simulink model "LPN_CVS_LVAD"  (R2014b)
settings: Solver=ode23s  StartTime=0.0  StopTime=15  FixedStep=0.01  RelTol=1e-2
values from neighbouring files (symbols this model uses):
  Cao = 0.08    [LPN_CVS_LVAD_Parameters.mat]
  Ccorat = 0.004    [LPN_CVS_LVAD_Parameters.mat]
  Ccorvn = 0.093    [LPN_CVS_LVAD_Parameters.mat]
  Cpa = 0.18    [LPN_CVS_LVAD_Parameters.mat]
  Cpart = 3.8    [LPN_CVS_LVAD_Parameters.mat]
  Cpvn = 20.5    [LPN_CVS_LVAD_Parameters.mat]
  CQao = 300    [LPN_CVS_LVAD_Parameters.mat]
  CQmi = 400    [LPN_CVS_LVAD_Parameters.mat]
  CQpa = 350    [LPN_CVS_LVAD_Parameters.mat]
  CQtri = 400    [LPN_CVS_LVAD_Parameters.mat]
  CsartLB = 1.9    [LPN_CVS_LVAD_Parameters.mat]
  CsartUB = 0.5    [LPN_CVS_LVAD_Parameters.mat]
  CsvnLB = 15    [LPN_CVS_LVAD_Parameters.mat]
  CsvnUB = 4    [LPN_CVS_LVAD_Parameters.mat]
  EedLA = 0.2125    [LPN_CVS_LVAD_Parameters.mat]
  EedRA = 0.1575    [LPN_CVS_LVAD_Parameters.mat]
  EmaxLA = 0.45    [LPN_CVS_LVAD_Parameters.mat]
  EmaxLV = 2.8    [LPN_CVS_LVAD_Parameters.mat]
  EmaxRA = 0.225    [LPN_CVS_LVAD_Parameters.mat]
  EmaxRV = 0.727    [LPN_CVS_LVAD_Parameters.mat]
  LV_Pd_alpha = 0.064    [LPN_CVS_LVAD_Parameters.mat]
  LV_Pd_beta = 2.5    [LPN_CVS_LVAD_Parameters.mat]
  LV_Pd_kappa = 0.033    [LPN_CVS_LVAD_Parameters.mat]
  Rao = 0.003    [LPN_CVS_LVAD_Parameters.mat]
  Rcorat = 26.25    [LPN_CVS_LVAD_Parameters.mat]
  Rcorvn = 8.75    [LPN_CVS_LVAD_Parameters.mat]
  Rpa = 0.002    [LPN_CVS_LVAD_Parameters.mat]
  Rpart = 0.31    [LPN_CVS_LVAD_Parameters.mat]
  Rpvn = 0.075    [LPN_CVS_LVAD_Parameters.mat]
  RsartLB = 2.3    [LPN_CVS_LVAD_Parameters.mat]
  RsartUB = 3.57    [LPN_CVS_LVAD_Parameters.mat]
  RsvnLB = 0.05    [LPN_CVS_LVAD_Parameters.mat]
  RsvnUB = 0.33    [LPN_CVS_LVAD_Parameters.mat]
  RV_Pd_alpha = 0.047    [LPN_CVS_LVAD_Parameters.mat]
  RV_Pd_beta = 2.5    [LPN_CVS_LVAD_Parameters.mat]
  RV_Pd_kappa = 0.028    [LPN_CVS_LVAD_Parameters.mat]
  V0ao = 112    [LPN_CVS_LVAD_Parameters.mat]
  V0ao_us = 101    [LPN_CVS_LVAD_Parameters.mat]
  V0corat = 6    [LPN_CVS_LVAD_Parameters.mat]
  V0corat_us = 5    [LPN_CVS_LVAD_Parameters.mat]
  V0corvn = 10    [LPN_CVS_LVAD_Parameters.mat]
  V0corvn_us = 9    [LPN_CVS_LVAD_Parameters.mat]
  V0LA = 22    [LPN_CVS_LVAD_Parameters.mat]
  V0LA_us = 5    [LPN_CVS_LVAD_Parameters.mat]
  V0LV = 95    [LPN_CVS_LVAD_Parameters.mat]
  V0LV_us = 5    [LPN_CVS_LVAD_Parameters.mat]
  V0pa = 78    [LPN_CVS_LVAD_Parameters.mat]
  V0pa_us = 77    [LPN_CVS_LVAD_Parameters.mat]
  V0part = 211    [LPN_CVS_LVAD_Parameters.mat]
  V0part_us = 91    [LPN_CVS_LVAD_Parameters.mat]
  V0pvn = 388    [LPN_CVS_LVAD_Parameters.mat]
  V0pvn_us = 168    [LPN_CVS_LVAD_Parameters.mat]
  V0RA = 20    [LPN_CVS_LVAD_Parameters.mat]
  V0RA_us = 5    [LPN_CVS_LVAD_Parameters.mat]
  V0RV = 125    [LPN_CVS_LVAD_Parameters.mat]
  V0RV_us = 10    [LPN_CVS_LVAD_Parameters.mat]
  V0sart_usLB = 91    [LPN_CVS_LVAD_Parameters.mat]
  V0sart_usUB = 39    [LPN_CVS_LVAD_Parameters.mat]
  V0sartLB = 301    [LPN_CVS_LVAD_Parameters.mat]
  V0sartUB = 87    [LPN_CVS_LVAD_Parameters.mat]
  V0svn_usLB = 385    [LPN_CVS_LVAD_Parameters.mat]
  V0svn_usUB = 165    [LPN_CVS_LVAD_Parameters.mat]
  V0svnLB = 477    [LPN_CVS_LVAD_Parameters.mat]
  V0svnUB = 220    [LPN_CVS_LVAD_Parameters.mat]
libraries: simulink x6
settings Model: Creator=Michael  LastModifiedBy=Michael
settings SolverCC: ZeroCrossAlgorithm=Adaptive
settings DataIOCC: MaxDataPoints=100

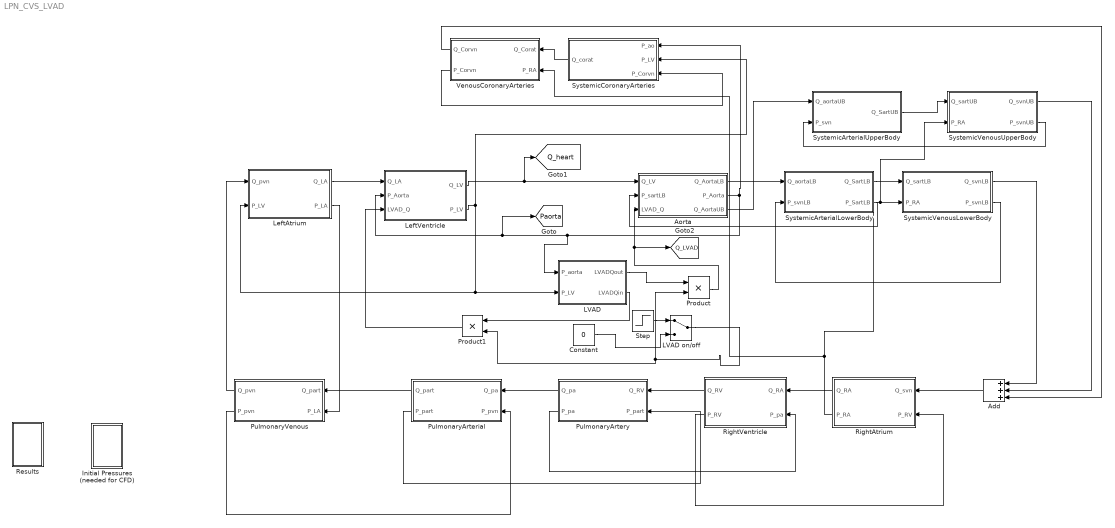
== system LPN_CVS_LVAD ==
  Add : Sum  Inputs=+++
  Aorta : Subsystem
  Constant : Constant  Value=0
  Initial Pressures (needed for CFD) : Subsystem
  LVAD : Subsystem
  LVAD on/off : ManualSwitch
  LeftAtrium : Subsystem
  LeftVentricle : Subsystem
  Product : Product
  Product1 : Product
  PulmonaryArterial : Subsystem
  PulmonaryArtery : Subsystem
  PulmonaryVenous : Subsystem
  Results : Subsystem
  RightAtrium : Subsystem
  RightVentricle : Subsystem
  Step : Step  Time=8  SampleTime=0
  SystemicArterialLowerBody : Subsystem
  SystemicArterialUpperBody : Subsystem
  SystemicCoronaryArteries : Subsystem
  SystemicVenousLowerBody : Subsystem
  SystemicVenousUpperBody : Subsystem
  VenousCoronaryArteries : Subsystem
  tag scope: Paorta=global, Q_LVAD=global, Q_heart=global
  wires:
  LeftVentricle/1(Q_LV) -> [Q_heart], Aorta/1(Q_LV)
  Aorta/1(Q_AortaLB) -> SystemicArterialLowerBody/1(Q_aortaLB)
  Aorta/2(P_Aorta) -> SystemicCoronaryArteries/1(P_ao), LVAD/1(P_aorta), [Paorta], LeftVentricle/2(P_Aorta)
  SystemicVenousLowerBody/2(P_svnLB) -> SystemicArterialLowerBody/2(P_svnLB)
  SystemicArterialLowerBody/1(Q_SartLB) -> SystemicVenousLowerBody/1(Q_sartLB)
  LeftAtrium/1(Q_LA) -> LeftVentricle/1(Q_LA)
  RightAtrium/1(Q_RA) -> RightVentricle/1(Q_RA)
  RightVentricle/1(Q_RV) -> PulmonaryArtery/1(Q_RV)
  PulmonaryArtery/2(P_pa) -> RightVentricle/2(P_pa)
  PulmonaryArterial/2(P_part) -> PulmonaryArtery/2(P_part)
  RightAtrium/2(P_RA) -> VenousCoronaryArteries/2(P_RA), SystemicVenousUpperBody/2(P_RA), SystemicVenousLowerBody/2(P_RA)
  PulmonaryArtery/1(Q_pa) -> PulmonaryArterial/1(Q_pa)
  PulmonaryArterial/1(Q_part) -> PulmonaryVenous/1(Q_part)
  PulmonaryVenous/2(P_pvn) -> PulmonaryArterial/2(P_pvn)
  LeftAtrium/2(P_LA) -> PulmonaryVenous/2(P_LA)
  PulmonaryVenous/1(Q_pvn) -> LeftAtrium/1(Q_pvn)
  SystemicArterialUpperBody/1(Q_SartUB) -> SystemicVenousUpperBody/1(Q_sartUB)
  SystemicVenousUpperBody/2(P_svnUB) -> SystemicArterialUpperBody/2(P_svn)
  Add/1 -> RightAtrium/1(Q_svn)
  SystemicVenousLowerBody/1(Q_svnLB) -> Add/1
  SystemicVenousUpperBody/1(Q_svnUB) -> Add/2
  SystemicArterialLowerBody/2(P_SartLB) -> Aorta/2(P_sartLB)
  Aorta/3(Q_AortaUB) -> SystemicArterialUpperBody/1(Q_aortaUB)
  RightVentricle/2(P_RV) -> RightAtrium/2(P_RV)
  LeftVentricle/2(P_LV) -> LVAD/2(P_LV), LeftAtrium/2(P_LV), SystemicCoronaryArteries/2(P_LV)
  SystemicCoronaryArteries/1(Q_corat) -> VenousCoronaryArteries/1(Q_Corat)
  VenousCoronaryArteries/2(P_Corvn) -> SystemicCoronaryArteries/3(P_Corvn)
  VenousCoronaryArteries/1(Q_Corvn) -> Add/3
  Constant/1 -> LVAD on/off/2
  Step/1 -> LVAD on/off/1
  LVAD/1(LVADQout) -> Product/1
  LVAD on/off/1 -> Product/2, Product1/2
  Product/1 -> [Q_LVAD], Aorta/3(LVAD_Q)
  Product1/1 -> LeftVentricle/3(LVAD_Q)
  LVAD/2("LVADQin ") -> Product1/1

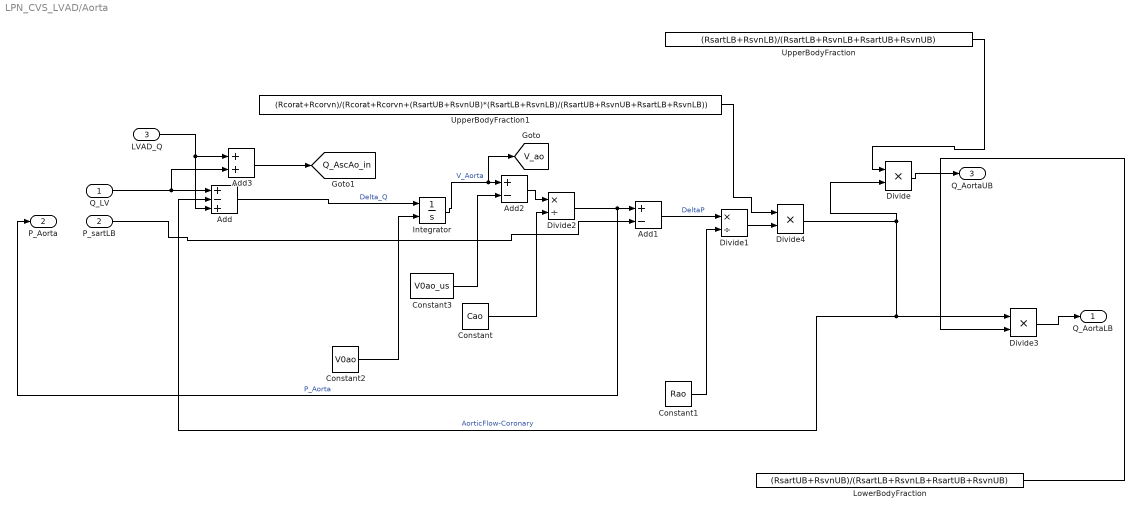
== system LPN_CVS_LVAD/Aorta ==
  Q_LV : Inport
  P_sartLB : Inport  Port=2
  LVAD_Q : Inport  Port=3
  Add : Sum  Inputs=+-+
  Add1 : Sum  Inputs=+-
  Add2 : Sum  Inputs=+-
  Add3 : Sum
  Constant : Constant  Value=Cao
  Constant1 : Constant  Value=Rao
  Constant2 : Constant  Value=V0ao
  Constant3 : Constant  Value=V0ao_us
  Divide : Product  Inputs=**
  Divide1 : Product  Inputs=*/
  Divide2 : Product  Inputs=*/
  Divide3 : Product  Inputs=**
  Divide4 : Product  Inputs=**
  Integrator : Integrator  InitialConditionSource=external
  LowerBodyFraction : Constant  Value=(RsartUB+RsvnUB)/(RsartLB+RsvnLB+RsartUB+RsvnUB)
  UpperBodyFraction : Constant  Value=(RsartLB+RsvnLB)/(RsartLB+RsvnLB+RsartUB+RsvnUB)
  UpperBodyFraction1 : Constant  Value=(Rcorat+Rcorvn)/(Rcorat+Rcorvn+(RsartUB+RsvnUB)*(RsartLB+RsvnLB)/(RsartUB+RsvnUB+RsartLB+RsvnLB))
  Q_AortaLB : Outport
  P_Aorta : Outport  Port=2
  Q_AortaUB : Outport  Port=3
  tag scope: Q_AscAo_in=global, V_ao=global
  wires:
  Add/1 -> Integrator/1  "Delta_Q"
  Constant1/1 -> Divide1/2
  Add1/1 -> Divide1/1  "DeltaP"
  Constant/1 -> Divide2/2
  P_sartLB/1 -> Add1/2
  Q_LV/1 -> Add3/2, Add/1
  Integrator/1 -> [V_ao], Add2/1  "V_Aorta"
  Constant2/1 -> Integrator/2
  Add2/1 -> Divide2/1
  Divide2/1 -> P_Aorta/1, Add1/1  "P_Aorta"
  Constant3/1 -> Add2/2
  Divide/1 -> Q_AortaUB/1
  Divide3/1 -> Q_AortaLB/1
  LowerBodyFraction/1 -> Divide3/2
  UpperBodyFraction/1 -> Divide/1
  UpperBodyFraction1/1 -> Divide4/1
  Divide1/1 -> Divide4/2
  Divide4/1 -> Add/2, Divide3/1, Divide/2  "AorticFlow-Coronary"
  LVAD_Q/1 -> Add3/1, Add/3
  Add3/1 -> [Q_AscAo_in]

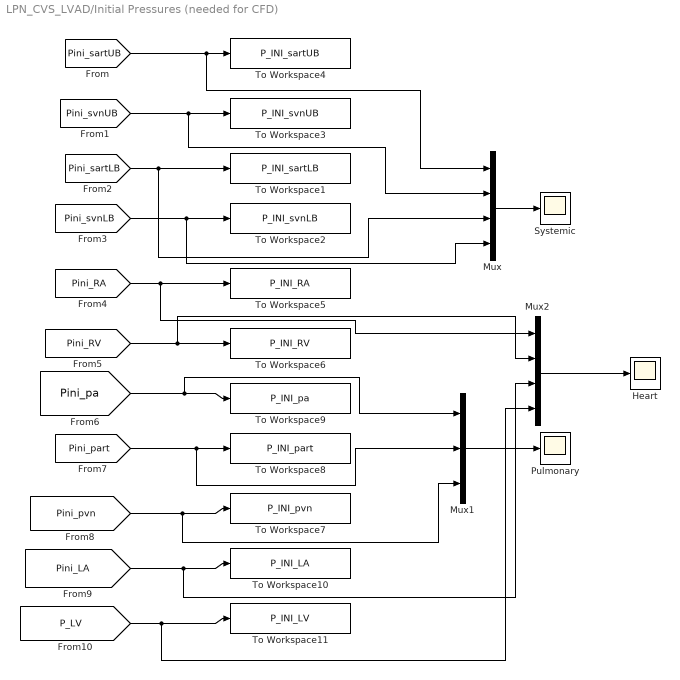
== system LPN_CVS_LVAD/Initial Pressures (needed for CFD) ==
  Heart : Scope
      settings: SaveName=ScopeData18
  Mux : Mux
  Mux1 : Mux  Inputs=3
  Mux2 : Mux
  Pulmonary : Scope
      settings: SaveName=ScopeData17
  Systemic : Scope
      settings: SaveName=ScopeData16
  To Workspace1 : ToWorkspace  VariableName=P_INI_sartLB  SampleTime=-1
  To Workspace10 : ToWorkspace  VariableName=P_INI_LA  SampleTime=-1
  To Workspace11 : ToWorkspace  VariableName=P_INI_LV  SampleTime=-1
  To Workspace2 : ToWorkspace  VariableName=P_INI_svnLB  SampleTime=-1
  To Workspace3 : ToWorkspace  VariableName=P_INI_svnUB  SampleTime=-1
  To Workspace4 : ToWorkspace  VariableName=P_INI_sartUB  SampleTime=-1
  To Workspace5 : ToWorkspace  VariableName=P_INI_RA  SampleTime=-1
  To Workspace6 : ToWorkspace  VariableName=P_INI_RV  SampleTime=-1
  To Workspace7 : ToWorkspace  VariableName=P_INI_pvn  SampleTime=-1
  To Workspace8 : ToWorkspace  VariableName=P_INI_part  SampleTime=-1
  To Workspace9 : ToWorkspace  VariableName=P_INI_pa  SampleTime=-1
  wires:
  [Pini_sartUB] -> Mux/1, To Workspace4/1
  [Pini_svnUB] -> Mux/2, To Workspace3/1
  [Pini_sartLB] -> Mux/3, To Workspace1/1
  [Pini_svnLB] -> Mux/4, To Workspace2/1
  [Pini_RA] -> Mux2/1, To Workspace5/1
  [Pini_RV] -> Mux2/2, To Workspace6/1
  [Pini_pa] -> Mux1/1, To Workspace9/1
  [Pini_part] -> Mux1/2, To Workspace8/1
  [Pini_pvn] -> Mux1/3, To Workspace7/1
  [Pini_LA] -> Mux2/3, To Workspace10/1
  [P_LV] -> Mux2/4, To Workspace11/1
  Mux1/1 -> Pulmonary/1
  Mux/1 -> Systemic/1
  Mux2/1 -> Heart/1

== system LPN_CVS_LVAD/LVAD ==
  P_aorta : Inport
  P_LV : Inport  Port=2
  Add2 : Sum  Inputs=+-
  Outlet Cannula : Subsystem
  PumpPerformance : Subsystem
  R_can_in : Gain  Gain=0.05
  Scope : Scope
      settings: SaveName=ScopeData24
  Scope1 : Scope
      settings: SaveName=ScopeData32
  LVADQout : Outport
  "LVADQin " : Outport  Port=2
  wires:
  P_aorta/1 -> Outlet Cannula/2(P_aorta)
  Outlet Cannula/2(LVADQout) -> LVADQout/1
  P_LV/1 -> Add2/1
  R_can_in/1 -> Add2/2
  PumpPerformance/1(LVADQin) -> Scope1/1, "LVADQin "/1, R_can_in/1, Outlet Cannula/1(LVADQin)
  Add2/1 -> PumpPerformance/1(P_can_in), Scope/1
  Outlet Cannula/1(P_can_out) -> PumpPerformance/2(P_can_out)

== system LPN_CVS_LVAD/LeftAtrium ==
  Q_pvn : Inport
  P_LV : Inport  Port=2
  Add : Sum  Inputs=+-
  Add2 : Sum  Inputs=+-
  AtrialElastance : Subsystem
  Constant2 : Constant  Value=V0LA
  Integrator : Integrator  InitialConditionSource=external
  Mitral Valve : Subsystem
  Product : Product
  Repeating Sequence : simulink/Sources/Repeating Sequence  rep_seq_t=time  rep_seq_y=e_a
  V0LA_US : Constant  Value=V0LA_us
  Q_LA : Outport
  P_LA : Outport  Port=2
  tag scope: Pini_LA=global, V_la=global
  wires:
  Q_pvn/1 -> Add2/1
  Add/1 -> Product/1
  V0LA_US/1 -> Add/2  "V0"
  Add2/1 -> Integrator/1  "Q_compliance"
  Integrator/1 -> [V_la], Add/1  "V_LV"
  Product/1 -> Mitral Valve/1(P_LA), [Pini_LA], P_LA/1  "P_LV(t)"
  Repeating Sequence/1 -> AtrialElastance/1(e_a)  "e_a"
  AtrialElastance/1(E(t)) -> Product/2
  Constant2/1 -> Integrator/2
  Mitral Valve/1(Q_LA) -> Q_LA/1, Add2/2
  P_LV/1 -> Mitral Valve/2(P_LV)

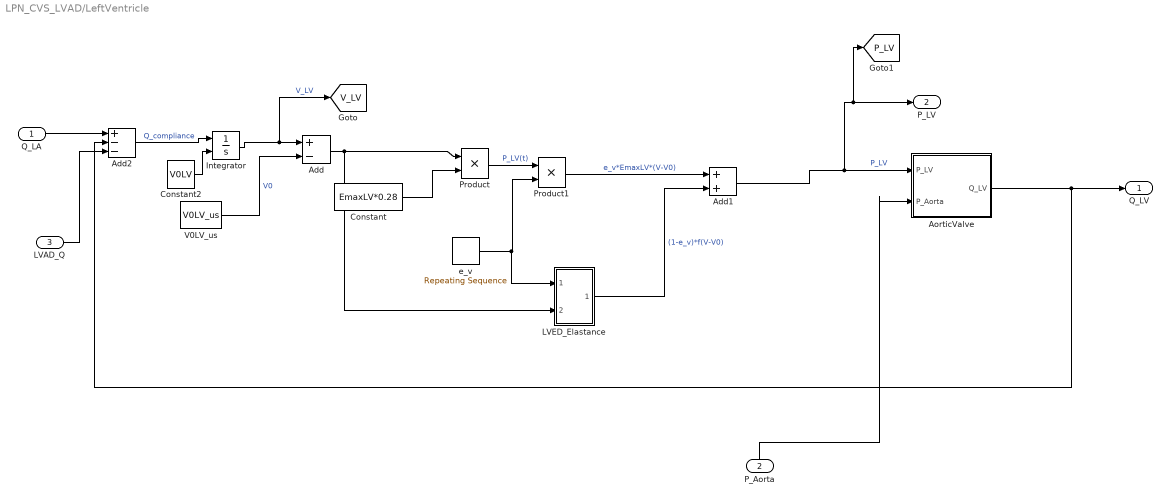
== system LPN_CVS_LVAD/LeftVentricle ==
  Q_LA : Inport
  P_Aorta : Inport  Port=2
  LVAD_Q : Inport  Port=3
  Add : Sum  Inputs=+-
  Add1 : Sum
  Add2 : Sum  Inputs=+--
  AorticValve : Subsystem
  Constant : Constant  Value=EmaxLV*0.28
  Constant2 : Constant  Value=V0LV
  Integrator : Integrator  InitialConditionSource=external
  LVED_Elastance : Subsystem
  Product : Product
  Product1 : Product
  V0LV_us : Constant  Value=V0LV_us
  e_v : simulink/Sources/Repeating Sequence  rep_seq_t=time  rep_seq_y=e_v
  Q_LV : Outport
  P_LV : Outport  Port=2
  tag scope: P_LV=global, V_LV=global
  wires:
  Q_LA/1 -> Add2/1
  Add/1 -> LVED_Elastance/2(V-V0), Product/1
  V0LV_us/1 -> Add/2  "V0"
  Add2/1 -> Integrator/1  "Q_compliance"
  Integrator/1 -> [V_LV], Add/1  "V_LV"
  Constant2/1 -> Integrator/2
  AorticValve/1(Q_LV) -> Add2/2, Q_LV/1
  P_Aorta/1 -> AorticValve/2(P_Aorta)
  Constant/1 -> Product/2
  Product/1 -> Product1/1  "P_LV(t)"
  e_v/1 -> LVED_Elastance/1(e_v), Product1/2
  Product1/1 -> Add1/1  "e_v*EmaxLV*(V-V0)"
  Add1/1 -> [P_LV], P_LV/1, AorticValve/1(P_LV)  "P_LV"
  LVED_Elastance/1(Eed) -> Add1/2  "(1-e_v)*f(V-V0)"
  LVAD_Q/1 -> Add2/3

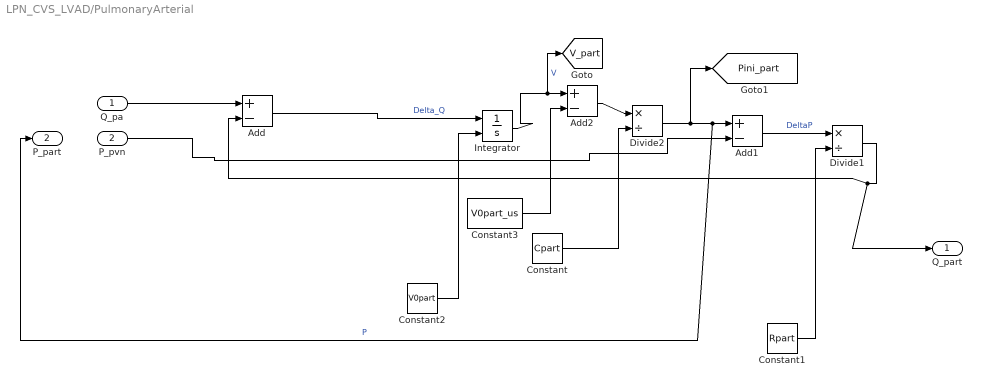
== system LPN_CVS_LVAD/PulmonaryArterial ==
  Q_pa : Inport
  P_pvn : Inport  Port=2
  Add : Sum  Inputs=+-
  Add1 : Sum  Inputs=+-
  Add2 : Sum  Inputs=+-
  Constant : Constant  Value=Cpart
  Constant1 : Constant  Value=Rpart
  Constant2 : Constant  Value=V0part
  Constant3 : Constant  Value=V0part_us
  Divide1 : Product  Inputs=*/
  Divide2 : Product  Inputs=*/
  Integrator : Integrator  InitialConditionSource=external
  Q_part : Outport
  P_part : Outport  Port=2
  tag scope: Pini_part=global, V_part=global
  wires:
  Divide1/1 -> Add/2, Q_part/1
  Add/1 -> Integrator/1  "Delta_Q"
  Constant1/1 -> Divide1/2
  Add1/1 -> Divide1/1  "DeltaP"
  Constant/1 -> Divide2/2
  P_pvn/1 -> Add1/2
  Q_pa/1 -> Add/1
  Integrator/1 -> [V_part], Add2/1  "V"
  Constant2/1 -> Integrator/2
  Add2/1 -> Divide2/1
  Divide2/1 -> [Pini_part], P_part/1, Add1/1  "P"
  Constant3/1 -> Add2/2

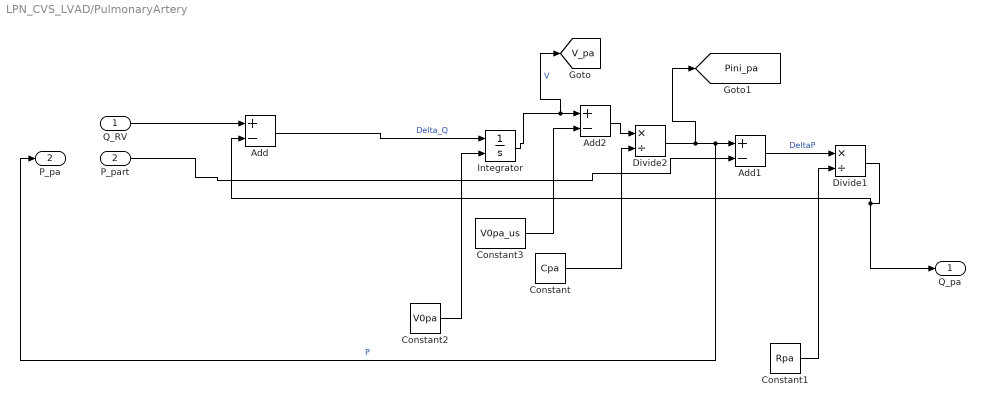
== system LPN_CVS_LVAD/PulmonaryArtery ==
  Q_RV : Inport
  P_part : Inport  Port=2
  Add : Sum  Inputs=+-
  Add1 : Sum  Inputs=+-
  Add2 : Sum  Inputs=+-
  Constant : Constant  Value=Cpa
  Constant1 : Constant  Value=Rpa
  Constant2 : Constant  Value=V0pa
  Constant3 : Constant  Value=V0pa_us
  Divide1 : Product  Inputs=*/
  Divide2 : Product  Inputs=*/
  Integrator : Integrator  InitialConditionSource=external
  Q_pa : Outport
  P_pa : Outport  Port=2
  tag scope: Pini_pa=global, V_pa=global
  wires:
  Divide1/1 -> Add/2, Q_pa/1
  Add/1 -> Integrator/1  "Delta_Q"
  Constant1/1 -> Divide1/2
  Add1/1 -> Divide1/1  "DeltaP"
  Constant/1 -> Divide2/2
  P_part/1 -> Add1/2
  Q_RV/1 -> Add/1
  Integrator/1 -> [V_pa], Add2/1  "V"
  Constant2/1 -> Integrator/2
  Add2/1 -> Divide2/1
  Divide2/1 -> [Pini_pa], P_pa/1, Add1/1  "P"
  Constant3/1 -> Add2/2

== system LPN_CVS_LVAD/PulmonaryVenous ==
  Q_part : Inport
  P_LA : Inport  Port=2
  Add : Sum  Inputs=+-
  Add1 : Sum  Inputs=+-
  Add2 : Sum  Inputs=+-
  Constant : Constant  Value=Cpvn
  Constant1 : Constant  Value=Rpvn
  Constant2 : Constant  Value=V0pvn
  Constant3 : Constant  Value=V0pvn_us  VectorParams1D=off
  Divide1 : Product  Inputs=*/
  Divide2 : Product  Inputs=*/
  Integrator : Integrator  InitialConditionSource=external
  Q_pvn : Outport
  P_pvn : Outport  Port=2
  tag scope: Pini_pvn=global, V_pvn=global
  wires:
  Divide1/1 -> Add/2, Q_pvn/1
  Add/1 -> Integrator/1  "Delta_Q"
  Constant1/1 -> Divide1/2
  Add1/1 -> Divide1/1  "DeltaP"
  Constant/1 -> Divide2/2
  P_LA/1 -> Add1/2
  Q_part/1 -> Add/1
  Integrator/1 -> [V_pvn], Add2/1  "V"
  Constant2/1 -> Integrator/2
  Add2/1 -> Divide2/1
  Divide2/1 -> [Pini_pvn], P_pvn/1, Add1/1  "P"
  Constant3/1 -> Add2/2

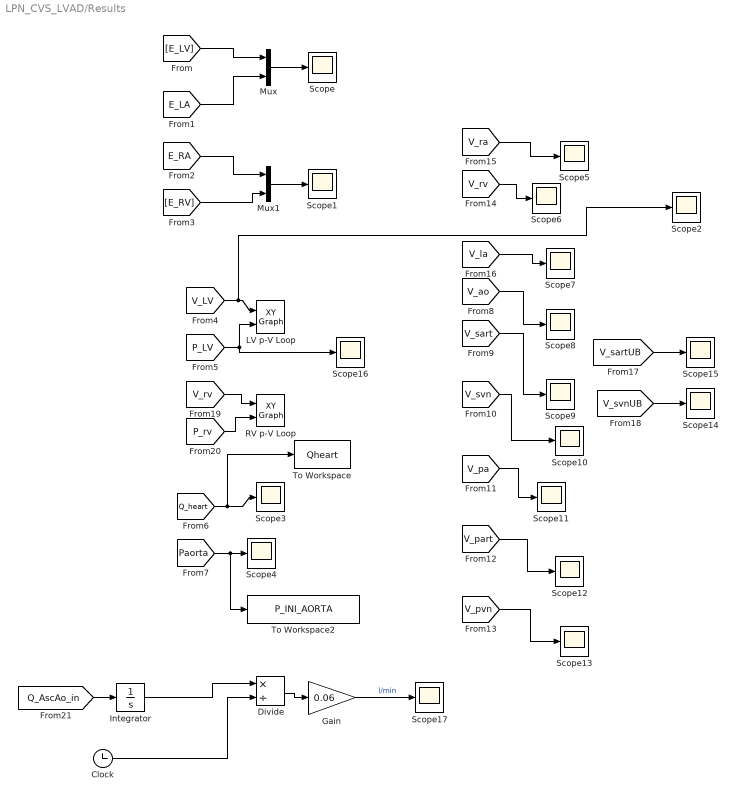
== system LPN_CVS_LVAD/Results ==
  Clock : Clock
  Divide : Product  Inputs=*/
  Gain : Gain  Gain=0.06
  Integrator : Integrator
  LV p-V Loop : simulink/Sinks/XY Graph  xmin=-1  xmax=200  ymin=-1  ymax=150  st=-1
  Mux : Mux  Inputs=2
  Mux1 : Mux  Inputs=2
  RV p-V Loop : simulink/Sinks/XY Graph  xmin=-1  xmax=150  ymin=-1  ymax=150  st=-1
  Scope{,1..17} (18 alike) : Scope
      Scope10 settings: SaveName=ScopeData12
      Scope11 settings: SaveName=ScopeData13
      Scope12 settings: YMin=240  YMax=330  SaveName=ScopeData14
      Scope13 settings: SaveName=ScopeData15
      Scope14 settings: SaveName=ScopeData21
      Scope15 settings: SaveName=ScopeData22
      Scope16 settings: SaveName=ScopeData20
      Scope17 settings: YMin=48  YMax=64  SaveName=ScopeData30
      Scope2 settings: SaveName=ScopeData4
      Scope3 settings: TimeRange=12.57889009793254  YMin=0  YMax=713.4020618556701  SaveName=ScopeData5
      Scope4 settings: SaveName=ScopeData6
      Scope5 settings: SaveName=ScopeData7
      Scope6 settings: SaveName=ScopeData8
      Scope7 settings: SaveName=ScopeData9
      Scope8 settings: SaveName=ScopeData10
      Scope9 settings: SaveName=ScopeData11
  To Workspace : ToWorkspace  VariableName=Qheart  SampleTime=-1
      settings: MaxDataPoints=100
  To Workspace2 : ToWorkspace  VariableName=P_INI_AORTA  SampleTime=-1
  wires:
  Mux1/1 -> Scope1/1
  Mux/1 -> Scope/1
  [E_LV] -> Mux/1
  [E_RA] -> Mux1/1
  [E_RV] -> Mux1/2
  [E_LA] -> Mux/2
  [V_LV] -> Scope2/1, LV p-V Loop/1
  [P_LV] -> LV p-V Loop/2, Scope16/1
  [Q_heart] -> To Workspace/1, Scope3/1
  [V_ra] -> Scope5/1
  [V_rv] -> Scope6/1
  [V_la] -> Scope7/1
  [V_ao] -> Scope8/1
  [V_sart] -> Scope9/1
  [V_svn] -> Scope10/1
  [V_pa] -> Scope11/1
  [V_part] -> Scope12/1
  [V_pvn] -> Scope13/1
  [V_svnUB] -> Scope14/1
  [V_sartUB] -> Scope15/1
  [V_rv] -> RV p-V Loop/1
  [P_rv] -> RV p-V Loop/2
  [Paorta] -> To Workspace2/1, Scope4/1
  Integrator/1 -> Divide/1
  Clock/1 -> Divide/2
  Divide/1 -> Gain/1
  [Q_AscAo_in] -> Integrator/1
  Gain/1 -> Scope17/1  "l/min"

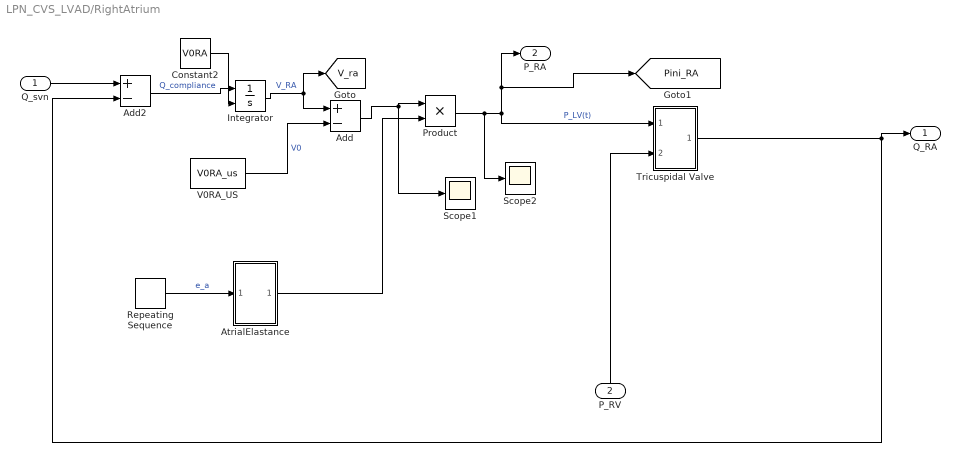
== system LPN_CVS_LVAD/RightAtrium ==
  Q_svn : Inport
  P_RV : Inport  Port=2
  Add : Sum  Inputs=+-
  Add2 : Sum  Inputs=+-
  AtrialElastance : Subsystem
  Constant2 : Constant  Value=V0RA
  Integrator : Integrator  InitialConditionSource=external
  Product : Product
  Repeating Sequence : simulink/Sources/Repeating Sequence  rep_seq_t=time  rep_seq_y=e_a
  Scope1 : Scope
      settings: SaveName=ScopeData2
  Scope2 : Scope
      settings: SaveName=ScopeData3
  Tricuspidal Valve : Subsystem
  V0RA_US : Constant  Value=V0RA_us
  Q_RA : Outport
  P_RA : Outport  Port=2
  tag scope: Pini_RA=global, V_ra=global
  wires:
  Q_svn/1 -> Add2/1
  Add/1 -> Product/1, Scope1/1
  V0RA_US/1 -> Add/2  "V0"
  Add2/1 -> Integrator/1  "Q_compliance"
  Integrator/1 -> [V_ra], Add/1  "V_RA"
  Product/1 -> Scope2/1, Tricuspidal Valve/1(P_RA), P_RA/1, [Pini_RA]  "P_LV(t)"
  Repeating Sequence/1 -> AtrialElastance/1(e_a)  "e_a"
  AtrialElastance/1(E(t)) -> Product/2
  Constant2/1 -> Integrator/2
  Tricuspidal Valve/1(Q_RV) -> Q_RA/1, Add2/2
  P_RV/1 -> Tricuspidal Valve/2(P_RV)

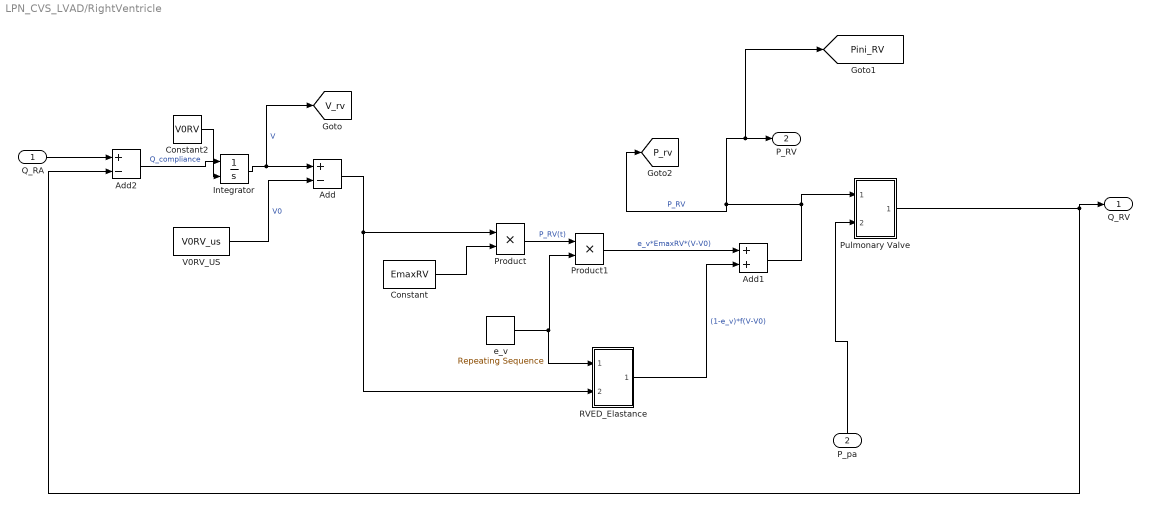
== system LPN_CVS_LVAD/RightVentricle ==
  Q_RA : Inport
  P_pa : Inport  Port=2
  Add : Sum  Inputs=+-
  Add1 : Sum
  Add2 : Sum  Inputs=+-
  Constant : Constant  Value=EmaxRV
  Constant2 : Constant  Value=V0RV
  Integrator : Integrator  InitialConditionSource=external
  Product : Product
  Product1 : Product
  Pulmonary Valve : Subsystem
  RVED_Elastance : Subsystem
  V0RV_US : Constant  Value=V0RV_us
  e_v : simulink/Sources/Repeating Sequence  rep_seq_t=time  rep_seq_y=e_v
  Q_RV : Outport
  P_RV : Outport  Port=2
  tag scope: P_rv=global, Pini_RV=global, V_rv=global
  wires:
  Q_RA/1 -> Add2/1
  V0RV_US/1 -> Add/2  "V0"
  Add2/1 -> Integrator/1  "Q_compliance"
  Integrator/1 -> [V_rv], Add/1  "V"
  Constant2/1 -> Integrator/2
  Pulmonary Valve/1(Q_RV) -> Q_RV/1, Add2/2
  P_pa/1 -> Pulmonary Valve/2(Ppa)
  Add/1 -> Product/1, RVED_Elastance/2(V-V0)
  Constant/1 -> Product/2
  Product/1 -> Product1/1  "P_RV(t)"
  e_v/1 -> RVED_Elastance/1(e_v), Product1/2
  Product1/1 -> Add1/1  "e_v*EmaxRV*(V-V0)"
  RVED_Elastance/1(Eed) -> Add1/2  "(1-e_v)*f(V-V0)"
  Add1/1 -> Pulmonary Valve/1(P_RV), [Pini_RV], P_RV/1, [P_rv]  "P_RV"

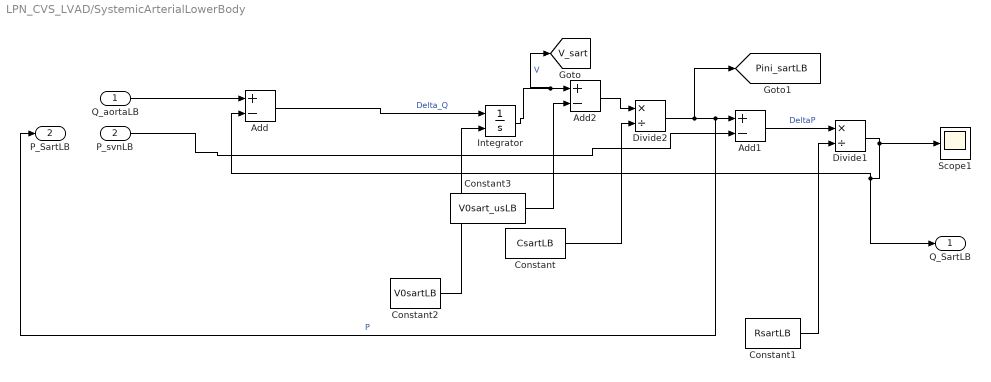
== system LPN_CVS_LVAD/SystemicArterialLowerBody ==
  Q_aortaLB : Inport
  P_svnLB : Inport  Port=2
  Add : Sum  Inputs=+-
  Add1 : Sum  Inputs=+-
  Add2 : Sum  Inputs=+-
  Constant : Constant  Value=CsartLB
  Constant1 : Constant  Value=RsartLB
  Constant2 : Constant  Value=V0sartLB
  Constant3 : Constant  Value=V0sart_usLB
  Divide1 : Product  Inputs=*/
  Divide2 : Product  Inputs=*/
  Integrator : Integrator  InitialConditionSource=external
  Scope1 : Scope
      settings: SaveName=ScopeData31
  Q_SartLB : Outport
  P_SartLB : Outport  Port=2
  tag scope: Pini_sartLB=global, V_sart=global
  wires:
  Divide1/1 -> Add/2, Q_SartLB/1, Scope1/1
  Add/1 -> Integrator/1  "Delta_Q"
  Constant1/1 -> Divide1/2
  Add1/1 -> Divide1/1  "DeltaP"
  Constant/1 -> Divide2/2
  P_svnLB/1 -> Add1/2
  Q_aortaLB/1 -> Add/1
  Integrator/1 -> [V_sart], Add2/1  "V"
  Constant2/1 -> Integrator/2
  Add2/1 -> Divide2/1
  Divide2/1 -> [Pini_sartLB], P_SartLB/1, Add1/1  "P"
  Constant3/1 -> Add2/2

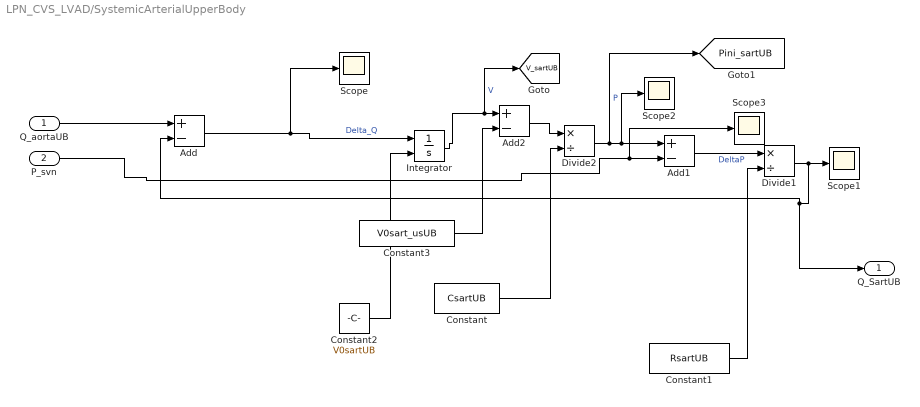
== system LPN_CVS_LVAD/SystemicArterialUpperBody ==
  Q_aortaUB : Inport
  P_svn : Inport  Port=2
  Add : Sum  Inputs=+-
  Add1 : Sum  Inputs=+-
  Add2 : Sum  Inputs=+-
  Constant : Constant  Value=CsartUB
  Constant1 : Constant  Value=RsartUB
  Constant2 : Constant  Value=V0sartUB
  Constant3 : Constant  Value=V0sart_usUB
  Divide1 : Product  Inputs=*/
  Divide2 : Product  Inputs=*/
  Integrator : Integrator  InitialConditionSource=external
  Scope{,1..3} (4 alike) : Scope
      Scope settings: SaveName=ScopeData26
      Scope1 settings: SaveName=ScopeData27
      Scope2 settings: SaveName=ScopeData28
      Scope3 settings: SaveName=ScopeData29
  Q_SartUB : Outport
  tag scope: Pini_sartUB=global, V_sartUB=global
  wires:
  Divide1/1 -> Add/2, Q_SartUB/1, Scope1/1
  Add/1 -> Scope/1, Integrator/1  "Delta_Q"
  Constant1/1 -> Divide1/2
  Add1/1 -> Divide1/1  "DeltaP"
  Constant/1 -> Divide2/2
  P_svn/1 -> Scope3/1, Add1/2
  Q_aortaUB/1 -> Add/1
  Integrator/1 -> [V_sartUB], Add2/1  "V"
  Constant2/1 -> Integrator/2
  Add2/1 -> Divide2/1
  Divide2/1 -> [Pini_sartUB], Scope2/1, Add1/1  "P"
  Constant3/1 -> Add2/2

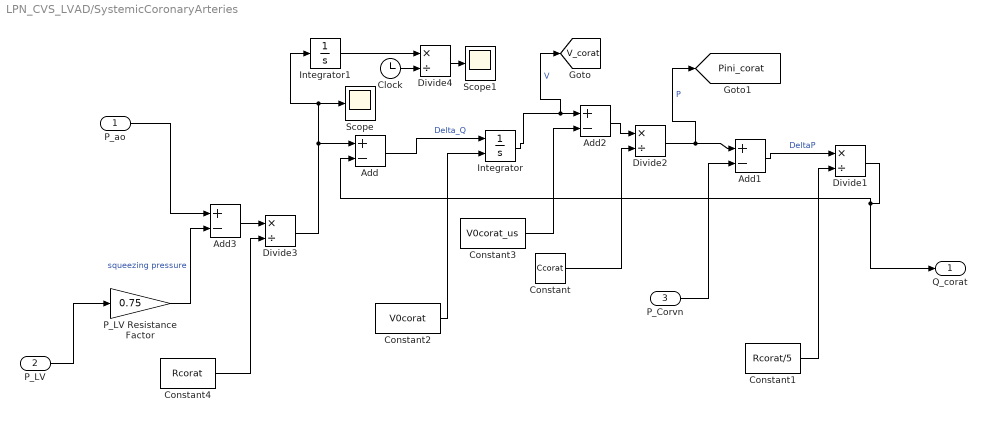
== system LPN_CVS_LVAD/SystemicCoronaryArteries ==
  P_ao : Inport
  P_LV : Inport  Port=2
  P_Corvn : Inport  Port=3
  Add{,1..3} (4 alike) : Sum  Inputs=+-
  Clock : Clock
  Constant : Constant  Value=Ccorat
  Constant1 : Constant  Value=Rcorat/5
  Constant2 : Constant  Value=V0corat
  Constant3 : Constant  Value=V0corat_us
  Constant4 : Constant  Value=Rcorat
  Divide{1..4} (4 alike) : Product  Inputs=*/
  Integrator : Integrator  InitialConditionSource=external
  Integrator1 : Integrator
  P_LV Resistance Factor : Gain  Gain=0.75
  Scope : Scope
      settings: YMin=-0.3  YMax=0  SaveName=ScopeData19
  Scope1 : Scope
      settings: YMin=-0.3  YMax=0  SaveName=ScopeData23
  Q_corat : Outport
  tag scope: Pini_corat=global, V_corat=global
  wires:
  Divide1/1 -> Add/2, Q_corat/1
  Add/1 -> Integrator/1  "Delta_Q"
  Constant1/1 -> Divide1/2
  Add1/1 -> Divide1/1  "DeltaP"
  Constant/1 -> Divide2/2
  P_LV/1 -> P_LV Resistance Factor/1
  Integrator/1 -> [V_corat], Add2/1  "V"
  Constant2/1 -> Integrator/2
  Add2/1 -> Divide2/1
  Divide2/1 -> [Pini_corat], Add1/1  "P"
  Constant3/1 -> Add2/2
  P_Corvn/1 -> Add1/2
  P_ao/1 -> Add3/1
  P_LV Resistance Factor/1 -> Add3/2  "squeezing pressure"
  Add3/1 -> Divide3/1
  Constant4/1 -> Divide3/2
  Divide3/1 -> Scope/1, Integrator1/1, Add/1
  Integrator1/1 -> Divide4/1
  Clock/1 -> Divide4/2
  Divide4/1 -> Scope1/1

== system LPN_CVS_LVAD/SystemicVenousLowerBody ==
  Q_sartLB : Inport
  P_RA : Inport  Port=2
  Add : Sum  Inputs=+-
  Add1 : Sum  Inputs=+-
  Add2 : Sum  Inputs=+-
  Constant : Constant  Value=CsvnLB
  Constant1 : Constant  Value=RsvnLB
  Constant2 : Constant  Value=V0svnLB
  Constant3 : Constant  Value=V0svn_usLB
  Divide1 : Product  Inputs=*/
  Divide2 : Product  Inputs=*/
  Integrator : Integrator  InitialConditionSource=external
  Q_svnLB : Outport
  P_svnLB : Outport  Port=2
  tag scope: Pini_svnLB=global, V_svn=global
  wires:
  Divide1/1 -> Add/2, Q_svnLB/1
  Add/1 -> Integrator/1  "Delta_Q"
  Constant1/1 -> Divide1/2
  Add1/1 -> Divide1/1  "DeltaP"
  Constant/1 -> Divide2/2
  P_RA/1 -> Add1/2
  Q_sartLB/1 -> Add/1
  Integrator/1 -> [V_svn], Add2/1  "V"
  Constant2/1 -> Integrator/2
  Add2/1 -> Divide2/1
  Divide2/1 -> [Pini_svnLB], P_svnLB/1, Add1/1  "P"
  Constant3/1 -> Add2/2

== system LPN_CVS_LVAD/SystemicVenousUpperBody ==
  Q_sartUB : Inport
  P_RA : Inport  Port=2
  Add : Sum  Inputs=+-
  Add1 : Sum  Inputs=+-
  Add2 : Sum  Inputs=+-
  Constant : Constant  Value=CsvnUB
  Constant1 : Constant  Value=RsvnUB
  Constant2 : Constant  Value=V0svnUB
  Constant3 : Constant  Value=V0svn_usUB
  Divide1 : Product  Inputs=*/
  Divide2 : Product  Inputs=*/
  Integrator : Integrator  InitialConditionSource=external
  Q_svnUB : Outport
  P_svnUB : Outport  Port=2
  tag scope: Pini_svnUB=global, V_svnUB=global
  wires:
  Divide1/1 -> Add/2, Q_svnUB/1
  Add/1 -> Integrator/1  "Delta_Q"
  Constant1/1 -> Divide1/2
  Add1/1 -> Divide1/1  "DeltaP"
  Constant/1 -> Divide2/2
  P_RA/1 -> Add1/2
  Q_sartUB/1 -> Add/1
  Integrator/1 -> [V_svnUB], Add2/1  "V"
  Constant2/1 -> Integrator/2
  Add2/1 -> Divide2/1
  Divide2/1 -> [Pini_svnUB], P_svnUB/1, Add1/1  "P"
  Constant3/1 -> Add2/2

== system LPN_CVS_LVAD/VenousCoronaryArteries ==
  Q_Corat : Inport
  P_RA : Inport  Port=2
  Add : Sum  Inputs=+-
  Add1 : Sum  Inputs=+-
  Add2 : Sum  Inputs=+-
  Constant : Constant  Value=Ccorvn
  Constant1 : Constant  Value=Rcorvn
  Constant2 : Constant  Value=V0corvn
  Constant3 : Constant  Value=V0corvn_us
  Divide1 : Product  Inputs=*/
  Divide2 : Product  Inputs=*/
  Integrator : Integrator  InitialConditionSource=external
  Q_Corvn : Outport
  P_Corvn : Outport  Port=2
  tag scope: Pini_corvn=global, V_corvn=global
  wires:
  Divide1/1 -> Add/2, Q_Corvn/1
  Add/1 -> Integrator/1  "Delta_Q"
  Constant1/1 -> Divide1/2
  Add1/1 -> Divide1/1  "DeltaP"
  Constant/1 -> Divide2/2
  Q_Corat/1 -> Add/1
  Integrator/1 -> [V_corvn], Add2/1  "V"
  Constant2/1 -> Integrator/2
  Add2/1 -> Divide2/1
  Divide2/1 -> [Pini_corvn], P_Corvn/1, Add1/1  "P"
  Constant3/1 -> Add2/2
  P_RA/1 -> Add1/2

== system LPN_CVS_LVAD/LVAD/Outlet Cannula ==
  note: P
  LVADQin : Inport
  P_aorta : Inport  Port=2
  Add2 : Sum  Inputs=+-
  Add3 : Sum  Inputs=+-
  C_can_out : Constant  Value=0.1
  Divide1 : Product  Inputs=*/
  Divide2 : Product  Inputs=*/
  Integrator : Integrator  InitialConditionSource=external
  R_can_out : Constant  Value=0.05
  V0can : Constant  Value=13
  P_can_out : Outport
  LVADQout : Outport  Port=2
  wires:
  Divide1/1 -> Add2/2, LVADQout/1
  Add3/1 -> Divide1/1
  Integrator/1 -> Divide2/1
  R_can_out/1 -> Divide1/2
  V0can/1 -> Integrator/2
  LVADQin/1 -> Add2/1
  Add2/1 -> Integrator/1
  P_aorta/1 -> Add3/2
  C_can_out/1 -> Divide2/2
  Divide2/1 -> P_can_out/1, Add3/1

== system LPN_CVS_LVAD/LVAD/PumpPerformance ==
  P_can_in : Inport
  P_can_out : Inport  Port=2
  Add : Sum  Inputs=+-
  Add1 : Sum  Inputs=+-
  Product : Product  Inputs=**
  Scope1 : Scope
      settings: TimeRange=5  YMax=45  SaveName=ScopeData25
  a : Constant  Value=15
  b : Constant  Value=-0.2
  l/min=>ml/s : Gain  Gain=16.67
  LVADQin : Outport
  wires:
  P_can_in/1 -> Add1/1
  Add/1 -> l/min=>ml/s/1
  b/1 -> Product/2
  a/1 -> Add/1
  Add1/1 -> Product/1  "deltaP"
  Product/1 -> Scope1/1, Add/2
  l/min=>ml/s/1 -> LVADQin/1
  P_can_out/1 -> Add1/2

== system LPN_CVS_LVAD/LeftAtrium/AtrialElastance ==
  e_a : Inport
  Add1 : Sum  Inputs=+-
  Add2 : Sum
  Constant : Constant  Value=EmaxLA
  Constant1 : Constant  Value=EedLA
  Product : Product
  E(t) : Outport
  tag scope: E_LA=global
  wires:
  e_a/1 -> Product/1
  Constant/1 -> Add1/1
  Product/1 -> Add2/1
  Constant1/1 -> Add1/2, Add2/2
  Add2/1 -> E(t)/1, [E_LA]
  Add1/1 -> Product/2

== system LPN_CVS_LVAD/LeftAtrium/Mitral Valve ==
  P_LA : Inport
  P_LV : Inport  Port=2
  Add1 : Sum  Inputs=+-
  Product1 : Product
  Rvalve : Constant  Value=CQmi
  Sqrt : Sqrt  SaturateOnIntegerOverflow=on
  ValveDiode1 : Saturate  UpperLimit=inf  LowerLimit=0.0001  ZeroCross=off
  Q_LA : Outport
  wires:
  P_LV/1 -> Add1/2
  Add1/1 -> ValveDiode1/1  "Delta_P"
  P_LA/1 -> Add1/1
  ValveDiode1/1 -> Sqrt/1
  Rvalve/1 -> Product1/2
  Sqrt/1 -> Product1/1
  Product1/1 -> Q_LA/1  "Q_LA"

== system LPN_CVS_LVAD/LeftVentricle/AorticValve ==
  P_LV : Inport
  P_Aorta : Inport  Port=2
  Add1 : Sum  Inputs=+-
  Product1 : Product
  Rvalve : Constant  Value=CQao
  Scope : Scope
      settings: SaveName=ScopeData34
  Sqrt : Sqrt  SaturateOnIntegerOverflow=on
  ValveDiode : Saturate  UpperLimit=inf  LowerLimit=0  ZeroCross=off
  Q_LV : Outport
  wires:
  P_Aorta/1 -> Add1/2
  Add1/1 -> Scope/1, ValveDiode/1  "Delta_P"
  ValveDiode/1 -> Sqrt/1
  Sqrt/1 -> Product1/1
  Product1/1 -> Q_LV/1  "Q_LV"
  Rvalve/1 -> Product1/2
  P_LV/1 -> Add1/1

== system LPN_CVS_LVAD/LeftVentricle/LVED_Elastance ==
  e_v : Inport
  V-V0 : Inport  Port=2
  Add : Sum  Inputs=+-
  Add1 : Sum
  Constant : Constant
  Math Function : Math  SaturateOnIntegerOverflow=on
  Pasym : Constant  Value=LV_Pd_beta
  Pinter : Constant  Value=LV_Pd_alpha
  Product : Product
  Product1 : Product
  Product2 : Product
  kappa : Constant  Value=LV_Pd_kappa
  Eed : Outport
  wires:
  e_v/1 -> Add/2
  Constant/1 -> Add/1
  Add/1 -> Product/1
  V-V0/1 -> Product1/1
  kappa/1 -> Product1/2
  Product1/1 -> Math Function/1
  Math Function/1 -> Product2/1
  Pinter/1 -> Product2/2
  Product2/1 -> Add1/1
  Pasym/1 -> Add1/2
  Product/1 -> Eed/1
  Add1/1 -> Product/2

== system LPN_CVS_LVAD/RightAtrium/AtrialElastance ==
  e_a : Inport
  Add : Sum
  Add1 : Sum  Inputs=+-
  Constant : Constant  Value=EmaxRA
  Constant1 : Constant  Value=EedRA
  Product : Product
  E(t) : Outport
  tag scope: E_RA=global
  wires:
  e_a/1 -> Product/1
  Constant/1 -> Add1/1
  Product/1 -> Add/1
  Constant1/1 -> Add1/2, Add/2
  Add/1 -> [E_RA], E(t)/1
  Add1/1 -> Product/2

== system LPN_CVS_LVAD/RightAtrium/Tricuspidal Valve ==
  P_RA : Inport
  P_RV : Inport  Port=2
  Add1 : Sum  Inputs=+-
  Product1 : Product
  Rvalve : Constant  Value=CQtri
  Sqrt : Sqrt  SaturateOnIntegerOverflow=on
  ValveDiode : Saturate  UpperLimit=inf  LowerLimit=0.001  ZeroCross=off
  Q_RV : Outport
  wires:
  P_RA/1 -> Add1/1
  Sqrt/1 -> Product1/1
  ValveDiode/1 -> Sqrt/1
  Add1/1 -> ValveDiode/1  "Delta_P"
  Rvalve/1 -> Product1/2
  P_RV/1 -> Add1/2
  Product1/1 -> Q_RV/1  "Q_RV"

== system LPN_CVS_LVAD/RightVentricle/Pulmonary Valve ==
  P_RV : Inport
  Ppa : Inport  Port=2
  Add1 : Sum  Inputs=+-
  Product1 : Product
  Rvalve : Constant  Value=CQpa
  Sqrt : Sqrt  SaturateOnIntegerOverflow=on
  ValveDiode1 : Saturate  UpperLimit=inf  LowerLimit=0.001  ZeroCross=off
  Q_RV : Outport
  wires:
  P_RV/1 -> Add1/1
  Rvalve/1 -> Product1/2
  Sqrt/1 -> Product1/1
  Product1/1 -> Q_RV/1  "Q_RV"
  Add1/1 -> ValveDiode1/1  "Delta_P"
  Ppa/1 -> Add1/2
  ValveDiode1/1 -> Sqrt/1

== system LPN_CVS_LVAD/RightVentricle/RVED_Elastance ==
  e_v : Inport
  V-V0 : Inport  Port=2
  Add : Sum  Inputs=+-
  Add1 : Sum
  Constant : Constant
  Math Function : Math  SaturateOnIntegerOverflow=on
  Pasym : Constant  Value=RV_Pd_beta
  Pinter : Constant  Value=RV_Pd_alpha
  Product : Product
  Product1 : Product
  Product2 : Product
  kappa : Constant  Value=RV_Pd_kappa
  Eed : Outport
  wires:
  e_v/1 -> Add/2
  Constant/1 -> Add/1
  Add/1 -> Product/1
  V-V0/1 -> Product1/1
  kappa/1 -> Product1/2
  Product1/1 -> Math Function/1
  Math Function/1 -> Product2/1
  Pinter/1 -> Product2/2
  Product2/1 -> Add1/1
  Pasym/1 -> Add1/2
  Product/1 -> Eed/1
  Add1/1 -> Product/2
